simulink model "Servo_Driver_Test"  (R2023b)
settings: Solver=ode3  StartTime=0.0  StopTime=inf  RelTol=1e-3  EnableMultiTasking=on
settings Model: FPTRunName=Active  ExtModeTrigDuration=2  Creator=Rafael  LastModifiedBy=Rafael
settings SolverCC: AlgebraicLoopSolver=TrustRegion  AutoInsertRateTranBlk=on
settings DataIOCC: LimitDataPoints=on  SaveFormat=Array
settings OptimizationCC: ExpressionDepthLimit=2147483647  LifeSpan=Inf  MaxStackSize=64
settings DebuggingCC: UnderspecifiedInitializationDetection=Classic  MergeDetectMultiDrivingBlocksExec=none  FcnCallInpInsideContextMsg=warning  UnconnectedInputMsg=warning  UnconnectedOutputMsg=warning  UnconnectedLineMsg=warning  AllowSymbolicDim=off  StateNameClashWarn=warning  SFUnexpectedBacktrackingDiag=warning  SFNoUnconditionalDefaultTransitionDiag=warning  SFExecutionAtInitializationDiag=none  ArithmeticOperatorsInVariantConditions=warning
settings HardwareCC: ProdBitPerPointer=32  ProdBitPerSizeT=32  ProdBitPerPtrDiffT=32  ProdLargestAtomicInteger=Long  ProdLargestAtomicFloat=Double  ProdWordSize=32  ProdHWDeviceType=ARM Compatible->ARM Cortex
settings ModelReferenceCC: EnableRefExpFcnMdlSchedulingChecks=on  PropagateSignalLabelsOutOfModel=off
settings SFSimCC: SimUseLocalCustomCode=off  CustomCodeUndefinedFunction=UseInterfaceOnly
settings RTWCC: Description=Embedded Coder  SystemTargetFile=ert.tlc  HardwareBoard=Arduino Due  TemplateMakefile=ert_default_tmf  GenerateReport=on  RTWVerbose=off  RTWUseLocalCustomCode=off  Toolchain=Arduino ARM  BuildConfiguration=Faster Runs  LaunchReport=on  DLArmComputeVersion=19.05
settings CodeAppCC: ForceParamTrailComments=on  OperatorAnnotations=on  StateflowObjectComments=on  MATLABSourceComments=on
settings ERTTargetCC: MultiwordLength=2048  ERTCustomFileBanners=off  SupportContinuousTime=on  SupportNonInlinedSFcns=on  RemoveResetFunc=off  SupportVariableSizeSignals=on  ModelStepFunctionPrototypeControlCompliant=off  ExtModeTransport=3  ExtModeStaticAlloc=on  ExtModeStaticAllocSize=24576  ExtModeMexFile=ext_xcp  ExtModeIntrfLevel=Level2 - Open
settings ConfigComp: CovMetricSettings=dw  CovSaveCumulativeToWorkspaceVar=on  CovSaveSingleToWorkspaceVar=on  CovExternalEMLEnable=off  CovSFcnEnable=off

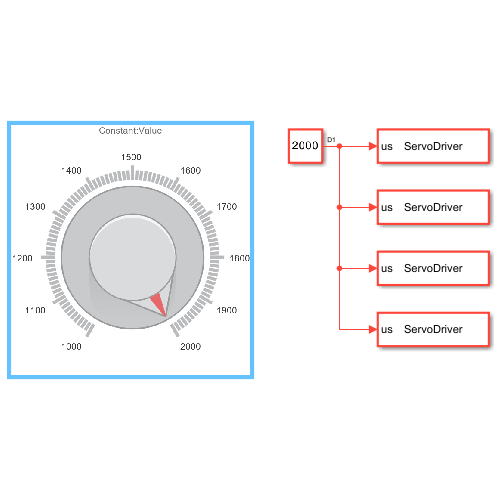
[thumbnail: Simulink's stored preview of the top-level diagram]
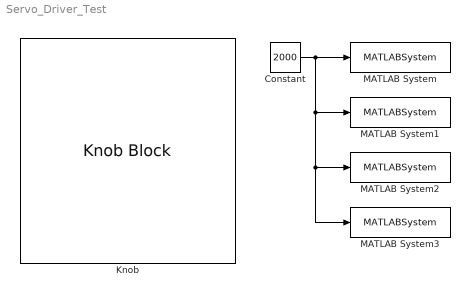
== system Servo_Driver_Test ==
  Constant : Constant  Value=2000  OutDataTypeStr=int32  SampleTime=1/50
  Knob : KnobBlock  ScaleMin=1000  ScaleMax=2000
  MATLAB System : MATLABSystem  System=ServoDriver  pin=8  min_us=1000  max_us=2000  SampleTime=1/50
      mask Type: ServoDriver
      mask Display:
      | disp('ServoDriver');
      | port_label('input',1,'us');
  MATLAB System1 : MATLABSystem  System=ServoDriver  pin=9  min_us=1000  max_us=2000  SampleTime=1/50
      mask Type: ServoDriver
      mask Display:
      | disp('ServoDriver');
      | port_label('input',1,'us');
  MATLAB System2 : MATLABSystem  System=ServoDriver  pin=10  min_us=1000  max_us=2000  SampleTime=1/50
      mask Type: ServoDriver
      mask Display:
      | disp('ServoDriver');
      | port_label('input',1,'us');
  MATLAB System3 : MATLABSystem  System=ServoDriver  pin=11  min_us=1000  max_us=2000  SampleTime=1/50
      mask Type: ServoDriver
      mask Display:
      | disp('ServoDriver');
      | port_label('input',1,'us');
  wires:
  Constant/1 -> MATLAB System1/1, MATLAB System2/1, MATLAB System3/1, MATLAB System/1
